simulink model "lab2_1"  (R2023a)
settings: Solver=VariableStepAuto  StartTime=0.0  StopTime=10  RelTol=1e-3
undefined symbols (not defined in the file or in its folder): u0, x10, x20, x30
settings Model: Creator=bz  LastModifiedBy=bz

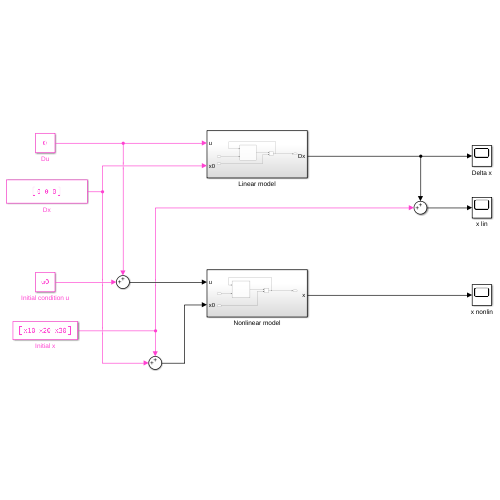
[thumbnail: Simulink's stored preview of the top-level diagram]
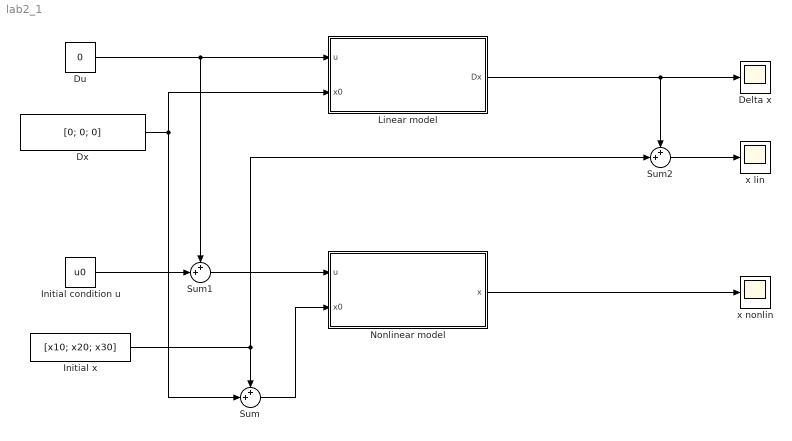
== system lab2_1 ==
  Delta x : Scope
  Du : Constant  Value=0
  Dx : Constant  Value=[0; 0; 0]
  Initial condition u : Constant  Value=u0
  Initial x : Constant  Value=[x10; x20; x30]
  Linear model : Subsystem
  Nonlinear model : Subsystem
  Sum : Sum  Inputs=++|
  Sum1 : Sum  Inputs=++|
  Sum2 : Sum  Inputs=++|
  x lin : Scope
  x nonlin : Scope
  wires:
  Dx/1 -> Sum/2, Linear model/2(x0)
  Du/1 -> Sum1/1, Linear model/1(u)
  Initial x/1 -> Sum/1, Sum2/2
  Initial condition u/1 -> Sum1/2
  Sum2/1 -> x lin/1
  Linear model/1(Dx) -> Delta x/1, Sum2/1
  Sum1/1 -> Nonlinear model/1(u)
  Sum/1 -> Nonlinear model/2(x0)
  Nonlinear model/1(x) -> x nonlin/1

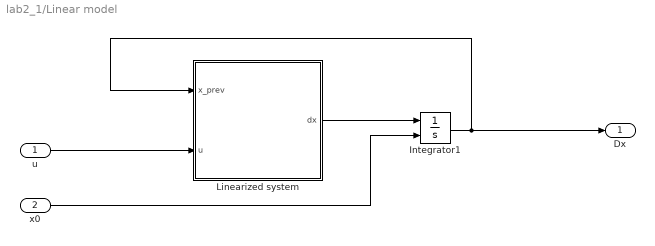
== system lab2_1/Linear model ==
  u : Inport
  x0 : Inport  Port=2
  Integrator1 : Integrator  InitialConditionSource=external
  Linearized system : MATLAB Function  TreatAsAtomicUnit=on
  Dx : Outport
  wires:
  Linearized system/1(dx) -> Integrator1/1
  Integrator1/1 -> Dx/1, Linearized system/1(x_prev)
  x0/1 -> Integrator1/2
  u/1 -> Linearized system/2(u)

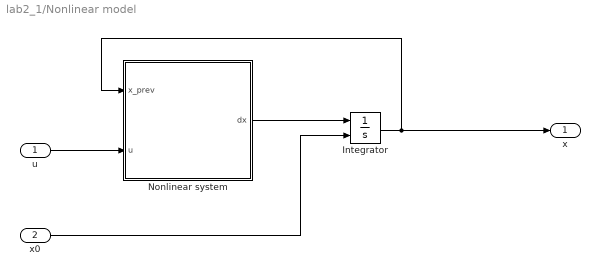
== system lab2_1/Nonlinear model ==
  u : Inport
  x0 : Inport  Port=2
  Integrator : Integrator  InitialConditionSource=external
  Nonlinear system : MATLAB Function  TreatAsAtomicUnit=on
  x : Outport
  wires:
  Integrator/1 -> x/1, Nonlinear system/1(x_prev)
  Nonlinear system/1(dx) -> Integrator/1
  x0/1 -> Integrator/2
  u/1 -> Nonlinear system/2(u)

== matlab function lab2_1/Nonlinear model/Nonlinear system ==
  data: x_prev input; u input; dx output size=[3,1]
function dx  = fcn(x_prev, u)

% x_prev
x1 = x_prev(1);
if x1 < 0
    x1 = 0;
end
x2 = x_prev(2);
x3 = x_prev(3);

FemP1 = 0.017521;
FemP2 = 0.0058231;

ci = -0.4;
ki = 4.4;
m = 0.016;
g = 9.81;

fiP1 = 1.4142e-4;
fiP2 = 4.5626e-3;

% fi = (fiP1/fiP2 * exp(-x1/fiP2));
% Fem1 = x3 ^ 2 * FemP1/FemP2 * exp(-x1/FemP2);

% x1_dot = 1;
% x2_dot = -Fem1/(2 * m) + g;
% x3_dot = 1/fi * (ki * u + ci - x3);

x1_dot = x2;
x2_dot = -(x3^2)*(FemP1/(FemP2*2*m))*exp(-x1/FemP2)+g;
x3_dot = 1/((fiP1/fiP2)*exp(-x1/fiP2))*(ki*u+ci-x3);

if x1_dot < 0
    x1_dot = 0;
end

% exp(-x1/FemP2)

dx = [x1_dot; x2_dot; x3_dot];

end

== matlab function lab2_1/Linear model/Linearized system ==
  data: x_prev input; u input; dx output size=[3,1]
function dx  = fcn(x_prev, u)
A = [0              0.0010      0;
     1.6847         0           -0.0257;
     0              0           -0.2888] * 1e3;

B = [0;
     0;
     1.2706] * 1e3;

dx = A * x_prev + B * u;

end
